simulink model "test_yL_epsL"  (Simulink 7.9)
settings: Solver=ode23  StartTime=0.0  StopTime=tend  FixedStep=0.01  RelTol=1e-3
values from neighbouring files (symbols this model uses):
  delta = @(u) 0.0015*(u-t0)*(u>t0) - 0.0035*(u-t1)*(u>t1)    [test_yL_epsL_.m]
undefined symbols (not defined in the file or in its folder): pin
libraries: library x4, simulink x2, simulink_extras x1
settings Model: Creator=Georg  LastModifiedBy=georgnestlinger
settings OptimizationCC: InlineParams=on
settings DebuggingCC: SolverPrmCheckMsg=none  FcnCallInpInsideContextMsg=Use local settings  StrictBusMsg=Warning
settings GRTTargetCC: CombineOutputUpdateFcns=off  GRTInterface=on

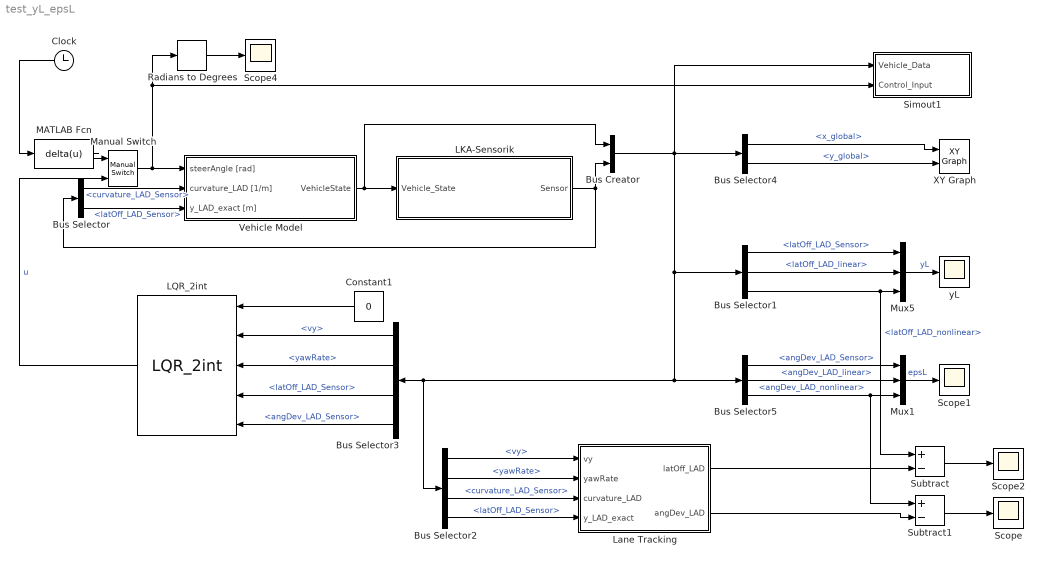
== system test_yL_epsL ==
  Bus Creator : BusCreator  Inputs=2
  Bus Selector : BusSelector  OutputSignals=curvature_LAD_Sensor,latOff_LAD_Sensor
  Bus Selector1 : BusSelector  OutputSignals=Sensor.latOff_LAD_Sensor,VehicleState.latOff_LAD_linear,VehicleState.latOff_LAD_nonlinear
  Bus Selector2 : BusSelector  OutputSignals=VehicleState.vy,VehicleState.yawRate,Sensor.curvature_LAD_Sensor,Sensor.latOff_LAD_Sensor
  Bus Selector3 : BusSelector  OutputSignals=VehicleState.vy,VehicleState.yawRate,Sensor.latOff_LAD_Sensor,Sensor.angDev_LAD_Sensor
  Bus Selector4 : BusSelector  OutputSignals=VehicleState.x_global,VehicleState.y_global
  Bus Selector5 : BusSelector  OutputSignals=Sensor.angDev_LAD_Sensor,VehicleState.angDev_LAD_linear,VehicleState.angDev_LAD_nonlinear
  Clock : Clock
  Constant1 : Constant  Value=0
  LKA-Sensorik : Subsystem  BlockChoice=Videosensorik
      settings: AttributesFormatString=%<BlockChoice>  TemplateBlock=library/LKA-Sensorik/LKA-Sensorik  MemberBlocks=Videosensorik
  LQR_2int : library/LKA-Controller/LQR_2int
  Lane Tracking : Subsystem
  MATLAB Fcn : MATLABFcn  MATLABFcn=delta(u)
  Manual Switch : simulink/Signal Routing/Manual Switch  sw=1  action=0  varsize=off
  Mux1 : Mux  Inputs=3
  Mux5 : Mux  Inputs=3
  Radians to Degrees : simulink_extras/Transformations/Radians to Degrees
  Scope{,1..2,4} (4 alike) : Scope
      Scope1 settings: SaveName=ScopeData2
      Scope2 settings: SaveName=ScopeData4
      Scope4 settings: YMin=-0.4  YMax=1.1
  Simout1 : Subsystem
  Subtract : Sum  Inputs=+-
  Subtract1 : Sum  Inputs=+-
  Vehicle Model : Subsystem
  XY Graph : simulink/Sinks/XY Graph  xmin=-50  xmax=700  ymin=-10  ymax=600  st=-1
  yL : Scope
      settings: TimeRange=28  YMin=-0.325  YMax=0  SaveName=ScopeData3
  wires:
  Bus Selector4/1 -> XY Graph/1  "<x_global>"
  Bus Selector4/2 -> XY Graph/2  "<y_global>"
  LKA-Sensorik/1(Sensor) -> Bus Creator/2, Bus Selector/1
  Bus Creator/1 -> Bus Selector4/1, Bus Selector1/1, Bus Selector3/1, Bus Selector2/1, Bus Selector5/1, Simout1/1(Vehicle_Data)
  Vehicle Model/1(VehicleState) -> Bus Creator/1, LKA-Sensorik/1(Vehicle_State)
  Constant1/1 -> LQR_2int/1
  Bus Selector3/1 -> LQR_2int/2  "<vy>"
  Bus Selector3/2 -> LQR_2int/3  "<yawRate>"
  Bus Selector3/3 -> LQR_2int/4  "<latOff_LAD_Sensor>"
  Bus Selector3/4 -> LQR_2int/5  "<angDev_LAD_Sensor>"
  LQR_2int/1 -> Manual Switch/2  "u"
  MATLAB Fcn/1 -> Manual Switch/1
  Manual Switch/1 -> Simout1/2(Control_Input), Radians to Degrees/1, Vehicle Model/1(steerAngle [rad])
  Bus Selector1/1 -> Mux5/1  "<latOff_LAD_Sensor>"
  Bus Selector1/2 -> Mux5/2  "<latOff_LAD_linear>"
  Clock/1 -> MATLAB Fcn/1
  Bus Selector2/2 -> Lane Tracking/2(yawRate)  "<yawRate>"
  Bus Selector2/1 -> Lane Tracking/1(vy)  "<vy>"
  Radians to Degrees/1 -> Scope4/1
  Bus Selector5/1 -> Mux1/1  "<angDev_LAD_Sensor>"
  Bus Selector5/2 -> Mux1/2  "<angDev_LAD_linear>"
  Bus Selector5/3 -> Mux1/3, Subtract1/1  "<angDev_LAD_nonlinear>"
  Bus Selector1/3 -> Mux5/3, Subtract/1  "<latOff_LAD_nonlinear>"
  Bus Selector2/3 -> Lane Tracking/3(curvature_LAD)  "<curvature_LAD_Sensor>"
  Lane Tracking/1(latOff_LAD) -> Subtract/2
  Lane Tracking/2(angDev_LAD) -> Subtract1/2
  Subtract1/1 -> Scope/1
  Mux1/1 -> Scope1/1  "epsL"
  Mux5/1 -> yL/1  "yL"
  Subtract/1 -> Scope2/1
  Bus Selector2/4 -> Lane Tracking/4(y_LAD_exact)  "<latOff_LAD_Sensor>"
  Bus Selector/1 -> Vehicle Model/2(curvature_LAD [1/m])  "<curvature_LAD_Sensor>"
  Bus Selector/2 -> Vehicle Model/3(y_LAD_exact [m])  "<latOff_LAD_Sensor>"

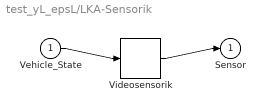
== system test_yL_epsL/LKA-Sensorik ==
  Vehicle_State : Inport
  Videosensorik : library/LKA-Sensorik/Videosensorik
  Sensor : Outport
  wires:
  Vehicle_State/1 -> Videosensorik/1
  Videosensorik/1 -> Sensor/1

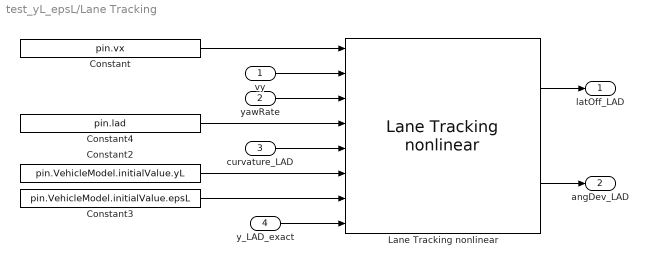
== system test_yL_epsL/Lane Tracking ==
  vy : Inport
  yawRate : Inport  Port=2
  curvature_LAD : Inport  Port=3
  y_LAD_exact : Inport  Port=4
  Constant : Constant  Value=pin.vx
  Constant2 : Constant  Value=pin.VehicleModel.initialValue.yL
  Constant3 : Constant  Value=pin.VehicleModel.initialValue.epsL
  Constant4 : Constant  Value=pin.lad
  Lane Tracking nonlinear : library/Vehicle Models/Lane Tracking/Lane Tracking nonlinear
  latOff_LAD : Outport
  angDev_LAD : Outport  Port=2
  wires:
  Constant/1 -> Lane Tracking nonlinear/1
  Constant4/1 -> Lane Tracking nonlinear/4
  Constant2/1 -> Lane Tracking nonlinear/6
  Constant3/1 -> Lane Tracking nonlinear/7
  vy/1 -> Lane Tracking nonlinear/2
  Lane Tracking nonlinear/1 -> latOff_LAD/1
  yawRate/1 -> Lane Tracking nonlinear/3
  curvature_LAD/1 -> Lane Tracking nonlinear/5
  Lane Tracking nonlinear/2 -> angDev_LAD/1
  y_LAD_exact/1 -> Lane Tracking nonlinear/8

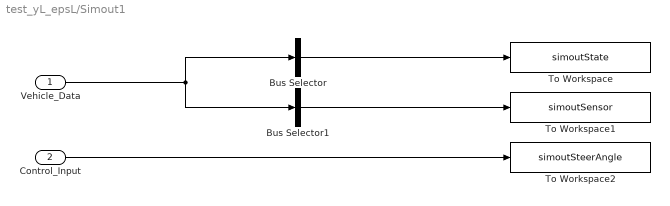
== system test_yL_epsL/Simout1 ==
  Vehicle_Data : Inport
  Control_Input : Inport  Port=2
  Bus Selector : BusSelector  OutputSignals=VehicleState  OutputAsBus=on
  Bus Selector1 : BusSelector  OutputSignals=Sensor  OutputAsBus=on
  To Workspace : ToWorkspace  VariableName=simoutState  SampleTime=-1  SaveFormat=Structure With Time
  To Workspace1 : ToWorkspace  VariableName=simoutSensor  SampleTime=-1  SaveFormat=Structure With Time
  To Workspace2 : ToWorkspace  VariableName=simoutSteerAngle  SampleTime=-1  SaveFormat=Structure With Time
  wires:
  Vehicle_Data/1 -> Bus Selector1/1, Bus Selector/1
  Control_Input/1 -> To Workspace2/1
  Bus Selector/1 -> To Workspace/1
  Bus Selector1/1 -> To Workspace1/1

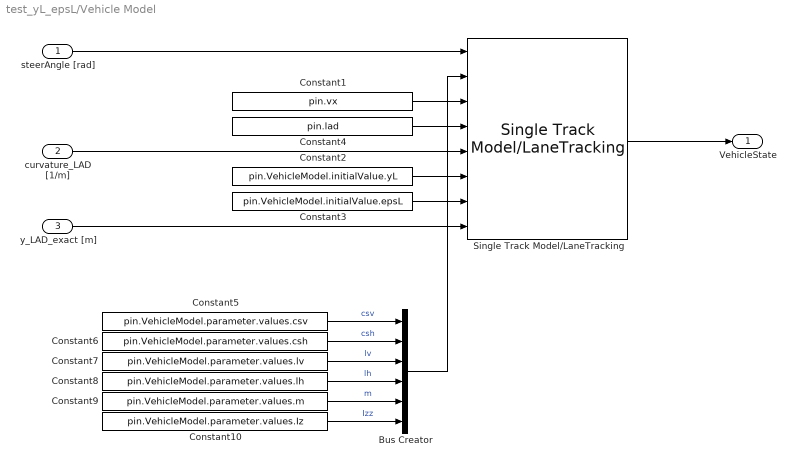
== system test_yL_epsL/Vehicle Model ==
  steerAngle [rad] : Inport
  curvature_LAD [1/m] : Inport  Port=2
  y_LAD_exact [m] : Inport  Port=3
  Bus Creator : BusCreator  Inputs=6
  Constant1 : Constant  Value=pin.vx
  Constant10 : Constant  Value=pin.VehicleModel.parameter.values.Iz
  Constant2 : Constant  Value=pin.VehicleModel.initialValue.yL
  Constant3 : Constant  Value=pin.VehicleModel.initialValue.epsL
  Constant4 : Constant  Value=pin.lad
  Constant5 : Constant  Value=pin.VehicleModel.parameter.values.csv
  Constant6 : Constant  Value=pin.VehicleModel.parameter.values.csh
  Constant7 : Constant  Value=pin.VehicleModel.parameter.values.lv
  Constant8 : Constant  Value=pin.VehicleModel.parameter.values.lh
  Constant9 : Constant  Value=pin.VehicleModel.parameter.values.m
  Single Track Model/LaneTracking : library/Vehicle Models/Single Track Model//LaneTracking
  VehicleState : Outport
  wires:
  Single Track Model/LaneTracking/1 -> VehicleState/1
  Constant2/1 -> Single Track Model/LaneTracking/6
  Constant3/1 -> Single Track Model/LaneTracking/7
  Constant1/1 -> Single Track Model/LaneTracking/3
  Constant4/1 -> Single Track Model/LaneTracking/4
  steerAngle [rad]/1 -> Single Track Model/LaneTracking/1
  curvature_LAD [1/m]/1 -> Single Track Model/LaneTracking/5
  y_LAD_exact [m]/1 -> Single Track Model/LaneTracking/8
  Constant5/1 -> Bus Creator/1  "csv"
  Constant6/1 -> Bus Creator/2  "csh"
  Constant7/1 -> Bus Creator/3  "lv"
  Constant8/1 -> Bus Creator/4  "lh"
  Constant9/1 -> Bus Creator/5  "m"
  Constant10/1 -> Bus Creator/6  "Izz"
  Bus Creator/1 -> Single Track Model/LaneTracking/2
